simulink model "main_quad_rev5_31_315pm"  (R2023a)
settings: Solver=FixedStepAuto  StartTime=0.0  StopTime=inf  FixedStep=0.005  RelTol=1e-3
libraries: canmsglib x16, speedgoatlib_IO691 x12, slrealtimeutilitieslib x8
(part 1 of 2)
settings Model: SimulationMode=external  NumberOfSteps=2  ExtModeEnableFloating=off  Creator=celwe  LastModifiedBy=johna
settings SolverCC: ConcurrentTasks=on  PositivePriorityOrder=on
settings OptimizationCC: BlockReduction=off  OptimizeBlockIOStorage=off
settings DebuggingCC: TasksWithSamePriorityMsg=none  UnconnectedInputMsg=warning  UnconnectedOutputMsg=warning  UnconnectedLineMsg=warning
settings HardwareCC: ProdBitPerLong=64  ProdLongLongMode=on  ProdHWDeviceType=Intel->x86-64 (Linux 64)
settings ModelReferenceCC: EnableRefExpFcnMdlSchedulingChecks=on
settings RTWCC: Description=Simulink Real-Time  SystemTargetFile=slrealtime.tlc  TemplateMakefile=slrealtime_default_tmf  Toolchain=Simulink Real-Time Toolchain  BuildConfiguration=Faster Runs  CodeExecutionProfiling=on  TargetLang=C++  DLArmComputeVersion=19.05

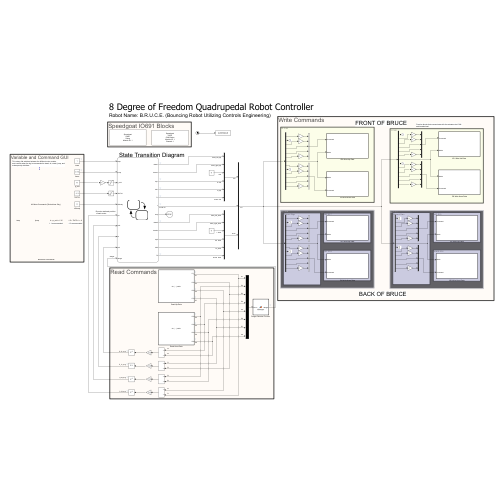
[thumbnail: Simulink's stored preview of the top-level diagram]
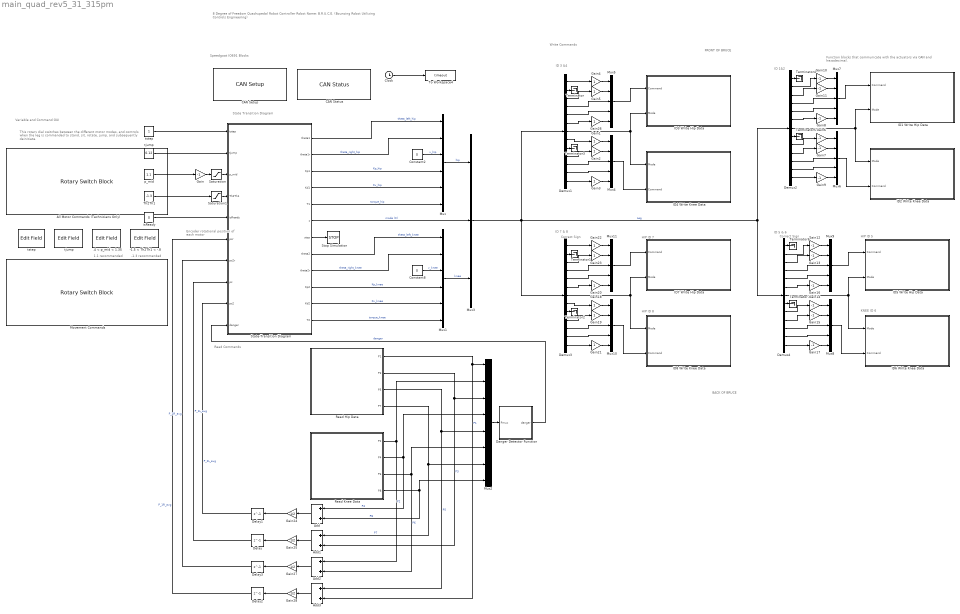
== system main_quad_rev5_31_315pm ==
  note: Variable and Command GUI
  note: 8 Degree of Freedom Quadrupedal Robot Controller
      | Robot Name: B.R.U.C.E. (Bouncing Robot Utilizing Controls Engineering)
  note: Encoder rotational position
      |  of each motor
  note: This rotary dial switches between the different motor modes,
      | and controls when the leg is commanded to stand, sit, rotate, jump, and
      | subsequently deinitiate.
  note: ID 1&2
  note: ID 3 &4
  note: BACK OF BRUCE
  note: HIP ID 5
  note: HIP ID 8
  note: KNEE ID 6
  note: ID 5 & 6
  note: FRONT OF BRUCE
  note: ID 7 & 8
  note: HIP ID 7
  note: Function blocks that communicate with the actuators via CAN
      | and hexadecimal.
  note: Correct Sign
  note: Correct Sign
  note: -1.3 recommended
  note: 1.1 recommended
  note: Speedgoat IO691 Blocks
  note: Read Commands
  note: Write Commands
  note: State Transition Diagram
  " tjump " : Constant  Value=0.12
  " tstep " : Constant
  -1.5 < Th2Th1 < -.8 : EditField  LabelPosition=Hide  ShowInitialText=on  Alignment=Center
  .4 < p_mid < 1.35 : EditField  LabelPosition=Hide  ShowInitialText=on  Alignment=Center
  Add{,1..3} (4 alike) : Sum
  "All Motor Commands (Technicians Only) " : RotarySwitchBlock
      settings: Values={{'Zeroing', 'Initiated', 'Stand', 'Sit', 'Right Up', 'Left Up', 'Jump', 'PrepJump', 'deinit'}, [0 1 2 3 5 6 7 8 4]}
  "CAN Setup " : speedgoatlib_IO691/Legacy/CAN Setup   moduletype=IO691  id=1  pciSlot=-1  chn1=CAN (HS)  chn2=CAN (HS)  chn3=Disabled  chn4=Disabled  initStruct=[]  termStruct=[]  ArbitrationbdrChn1=1.0 MBaud  ArbitrationManbdrChn1=[2,8,31,8]  FdbdrChn1=5.0 MBaud  FdManbdrChn1=[2,2,5,2]  ArbitrationbdrChn2=1.0 MBaud  ArbitrationManbdrChn2=[2,8,31,8]  FdbdrChn2=5.0 MBaud  FdManbdrChn2=[2,2,5,2]  ArbitrationbdrChn3=1.0 MBaud  ArbitrationManbdrChn3=[2,8,31,8]  FdbdrChn3=5.0 MBaud  FdManbdrChn3=[2,2,5,2]  ArbitrationbdrChn4=1.0 MBaud  ArbitrationManbdrChn4=[2,8,31,8]  FdbdrChn4=5.0 MBaud  FdManbdrChn4=[2,2,5,2]  moduleInitValues=[691 1 -1 -1]
      settings: SourceProductName=Simulink Real-Time: Speedgoat I/O Blockset
  CAN Status : speedgoatlib_IO691/Legacy/CAN Status  moduleId=1  sampleTime=-1  channel=1  busRecovery=Off  arrayOutput=off  controllerCpuLoad=off  controllerLiveCount=off  initModeAct=off  avgBusLoad=off  receiving=off  RxQueueEmpty=off  dataOverrunRcv=off  rxBufferLevel=off  txPending=off  dataOverrunTx=off  txBufferLevel=off  errWarnLimit=off  errPassLimit=off  errBusOff=off  busRecoveryCounter=off  busCouplingErr=off  transceiverErr=off  opMode=off  brp=off  timeSegment1=off  timeSegment2=off  synchronisationJumpWidth=off  dataTSEG1=off  dataTSEG2=off  dataSJW=off  moduleType=691  qtyStatBlk=1  ptIdx=0  isFDMod=0
      settings: SourceProductName=Simulink Real-Time: Speedgoat I/O Blockset
  Clock : Clock
  Constant2 : Constant  Value=0
  Constant8 : Constant  Value=0
  Danger Detector Function : MATLAB Function  TreatAsAtomicUnit=on
  Delay{,1..3} (4 alike) : Delay  DelayLength=1
  Demux{1..4} (4 alike) : Demux  Outputs=13
  Gain{,6..17} (13 alike) : Gain  Gain=-1
  Gain{1..5,18..23,26} (12 alike) : Gain
  Gain{24..25,27..28} (4 alike) : Gain  Gain=1/2
  ID1 Write Hip Data : Subsystem  TreatAsAtomicUnit=on
  ID2 Write Knee Data : Subsystem  TreatAsAtomicUnit=on
  ID3 Write Hip Data : Subsystem  TreatAsAtomicUnit=on
  ID4 Write Knee Data : Subsystem  TreatAsAtomicUnit=on
  ID5 Write Hip Data : Subsystem  TreatAsAtomicUnit=on
  ID6 Write Knee Data : Subsystem  TreatAsAtomicUnit=on
  ID7 Write Hip Data : Subsystem  TreatAsAtomicUnit=on
  ID8 Write Knee Data : Subsystem  TreatAsAtomicUnit=on
  Movement Commands : RotarySwitchBlock
      settings: Values={{'Stand', 'Sit', 'Right Up', 'Left Up', 'Jump', 'Prep Jump'}, [2 3 5 6 7 8]}
  Mux : Mux  Inputs=6
  Mux1 : Mux  Inputs=6
  Mux{4..11} (8 alike) : Mux  Inputs=5
  Mux2 : Mux  Inputs=8
  Mux3 : Mux  Inputs=3
  Read Hip Data : Subsystem  TreatAsAtomicUnit=on
  Read Knee Data : Subsystem  TreatAsAtomicUnit=on
  Saturation : Saturate  UpperLimit=-.4  LowerLimit=-1.35
  Saturation1 : Saturate  UpperLimit=-.8  LowerLimit=-1.5
  State-Transition Diagram : Stateflow chart  TreatAsAtomicUnit=on
      settings: PortSchema="{\"entries\":[{\"content\":{\"sides\":[{\"content\":{\"connectorIds\":[\"In7\",\"In8\",\"In9\",\"In10\",\"In4\",\"In5\",\"In6\",\"In1\",\"In2\",\"In3\"]},\"type\":\"ConnectorPlacement.EquallySpacedRectSide\",\"uuid\":\"09499f21-f50c-4ce4-914e-8b9942bcc246\"},{\"content\":{\"connectorIds\":[\"Out2\",\"Out11\",\"Out7\",\"Out9\",\"Out5\",\"Out4\",\"Out1\",\"Out3\",\"Out12\",\"Out8\",\"Out10\",\"Out6\"],\"side\":\"RIGHT\"},\"type\":\"ConnectorPlacement.EquallySpacedRectSide\",\"uuid\":\"b935e908-ace3-4dfb-ad6d-08dfed6ffdb3\"},{\"content\":{\"connectorIds\":[],\"side\":\"TOP\"},\"type\":\"ConnectorPlacement.EquallySpacedRectSide\",\"uuid\":\"4cd7c5d6-1f1f-4a1f-84b4-9b198395645e\"}]},\"type\":\"ConnectorPlacement.EquallySpacedConnector\",\"uuid\":\"2dc6a8af-05a8-4f21-87ab-6863f156f450\"}],\"packageUris\":[\"http://schema.mathworks.com/mf0/Connector/R2020b\"],\"version\":\"1.0\"}"
  Stop Simulation : Stop
  Terminator{,1..7} (8 alike) : Terminator
  Th2Th1 : Constant  Value=-1.3
  To Workspace4 : ToWorkspace  VariableName=timeout  SampleTime=-1
  isReady : Constant  Value=0
  p_mid : Constant  Value=1.1
  tjump : EditField  LabelPosition=Hide  ShowInitialText=on  Alignment=Center
  tstep : EditField  LabelPosition=Hide  ShowInitialText=on  Alignment=Center
  wires:
  Mux/1 -> Mux3/1  "hip"
  State-Transition Diagram/7(Kp1) -> Mux/4  "Kp_hip"
  State-Transition Diagram/5(T1) -> Mux/6  "torque_hip"
  Constant8/1 -> Mux1/3  "v_knee"
  Mux1/1 -> Mux3/3  "knee"
  State-Transition Diagram/4(c) -> Mux3/2  "mode (C)"
  Mux2/1 -> Danger Detector Function/1(Pmux)
  Danger Detector Function/1(danger) -> State-Transition Diagram/3(danger)  "danger"
  Delay/1 -> State-Transition Diagram/1(pc)  "P_1L_avg"
  State-Transition Diagram/1(stop) -> Stop Simulation/1
  Delay1/1 -> State-Transition Diagram/2(pc2)  "P_2L_avg"
  isReady/1 -> State-Transition Diagram/4(isReady)
  Clock/1 -> To Workspace4/1
  State-Transition Diagram/9(Kd1) -> Mux/5  "Kv_hip"
  Constant2/1 -> Mux/3  "v_hip"
  State-Transition Diagram/2(theta1) -> Mux/1  "theta_left_hip"
  Mux11/1 -> ID7 Write Hip Data/1(Command)
  Mux10/1 -> ID8 Write Knee Data/2(Command)
  Mux3/1 -> Demux3/1, Demux4/1, Demux2/1, Demux1/1  "Leg"
  Gain24/1 -> Delay1/1
  Gain25/1 -> Delay/1
  Add/1 -> Gain24/1
  Add1/1 -> Gain25/1
  Mux9/1 -> ID5 Write Hip Data/1(Command)
  Mux8/1 -> ID6 Write Knee Data/2(Command)
  Mux7/1 -> ID1 Write Hip Data/1(Command)
  Mux6/1 -> ID2 Write Knee Data/2(Command)
  Demux1/8 -> Gain1/1
  Demux1/5 -> Mux5/4
  Demux1/7 -> ID4 Write Knee Data/1(Mode), ID3 Write Hip Data/2(Mode)
  Demux1/12 -> Mux4/4
  Gain3/1 -> Mux4/5
  Gain1/1 -> Mux4/1
  Gain2/1 -> Mux4/2
  Mux5/1 -> ID3 Write Hip Data/1(Command)
  Gain4/1 -> Mux5/1
  Gain5/1 -> Mux5/2
  Mux4/1 -> ID4 Write Knee Data/2(Command)
  Demux1/6 -> Gain26/1
  Demux1/11 -> Mux4/3
  Gain26/1 -> Mux5/5
  Demux1/3 -> Gain5/1
  Demux1/10 -> Gain2/1
  Demux1/1 -> Gain4/1
  Demux1/4 -> Mux5/3
  Read Knee Data/1(P2) -> Add2/1, Mux2/2  "P2"
  Read Knee Data/2(P4) -> Add/1, Mux2/4  "P4"
  Read Knee Data/3(P6) -> Add2/2, Mux2/6  "P6"
  Read Knee Data/4(P8) -> Add/2, Mux2/8  "P8"
  Read Hip Data/4(P7) -> Add1/1, Mux2/7  "P7"
  Read Hip Data/3(P5) -> Add3/1, Mux2/5  "P5"
  Read Hip Data/2(P3) -> Add1/2, Mux2/3  "P3"
  Read Hip Data/1(P1) -> Add3/2, Mux2/1  "P1"
  Gain28/1 -> Delay2/1
  Gain27/1 -> Delay3/1
  Add2/1 -> Gain27/1
  Add3/1 -> Gain28/1
  Delay3/1 -> State-Transition Diagram/6(pc2r)  "P_2R_avg"
  Delay2/1 -> State-Transition Diagram/5(pcr)  "P_1R_avg"
  State-Transition Diagram/11(theta1r) -> Mux/2  "theta_right_hip"
  Demux1/13 -> Gain3/1
  Demux2/7 -> ID1 Write Hip Data/2(Mode), ID2 Write Knee Data/1(Mode)
  Demux2/4 -> Mux7/3
  Demux2/10 -> Gain7/1
  Demux2/6 -> Gain8/1
  Demux2/5 -> Mux7/4
  Demux2/11 -> Mux6/3
  Demux2/3 -> Gain11/1
  Demux2/12 -> Mux6/4
  Gain11/1 -> Mux7/2
  Gain10/1 -> Mux7/1
  Gain7/1 -> Mux6/2
  Demux2/13 -> Gain9/1
  Gain9/1 -> Mux6/5
  Gain8/1 -> Mux7/5
  Gain6/1 -> Mux6/1
  Demux2/2 -> Gain10/1
  Demux2/9 -> Gain6/1
  Demux3/7 -> ID7 Write Hip Data/2(Mode), ID8 Write Knee Data/1(Mode)
  Demux3/4 -> Mux11/3
  Demux3/10 -> Gain19/1
  Demux3/6 -> Gain20/1
  Demux3/5 -> Mux11/4
  Demux3/11 -> Mux10/3
  Demux3/3 -> Gain23/1
  Demux3/12 -> Mux10/4
  Gain23/1 -> Mux11/2
  Demux3/1 -> Gain22/1
  Gain22/1 -> Mux11/1
  Gain19/1 -> Mux10/2
  Demux3/13 -> Gain21/1
  Gain21/1 -> Mux10/5
  Demux3/8 -> Gain18/1
  Gain20/1 -> Mux11/5
  Gain18/1 -> Mux10/1
  Demux4/5 -> Mux9/4
  Demux4/6 -> Gain16/1
  Demux4/10 -> Gain15/1
  Demux4/7 -> ID6 Write Knee Data/1(Mode), ID5 Write Hip Data/2(Mode)
  Demux4/2 -> Gain12/1
  Demux4/3 -> Gain13/1
  Demux4/9 -> Gain14/1
  Demux4/11 -> Mux8/3
  Gain12/1 -> Mux9/1
  Gain13/1 -> Mux9/2
  Gain17/1 -> Mux8/5
  Demux4/13 -> Gain17/1
  Gain14/1 -> Mux8/1
  Gain15/1 -> Mux8/2
  Demux4/12 -> Mux8/4
  Gain16/1 -> Mux9/5
  Demux4/4 -> Mux9/3
  Demux1/2 -> Terminator/1
  Demux3/2 -> Terminator1/1
  Demux3/9 -> Terminator2/1
  Demux1/9 -> Terminator3/1
  Demux2/1 -> Terminator4/1
  Demux2/8 -> Terminator5/1
  Demux4/1 -> Terminator6/1
  Demux4/8 -> Terminator7/1
  State-Transition Diagram/12(theta2r) -> Mux1/2  "theta_right_knee"
  State-Transition Diagram/3(theta2) -> Mux1/1  "theta_left_knee"
  State-Transition Diagram/10(Kd2) -> Mux1/5  "Kv_knee"
  State-Transition Diagram/6(T2) -> Mux1/6  "torque_knee"
  State-Transition Diagram/8(Kp2) -> Mux1/4  "Kp_knee"
  " tjump "/1 -> State-Transition Diagram/8(tjump)
  " tstep "/1 -> State-Transition Diagram/7(tstep)
  p_mid/1 -> Gain/1
  Saturation/1 -> State-Transition Diagram/9(p_mid)
  Gain/1 -> Saturation/1
  Th2Th1/1 -> Saturation1/1
  Saturation1/1 -> State-Transition Diagram/10(Th2Th1)

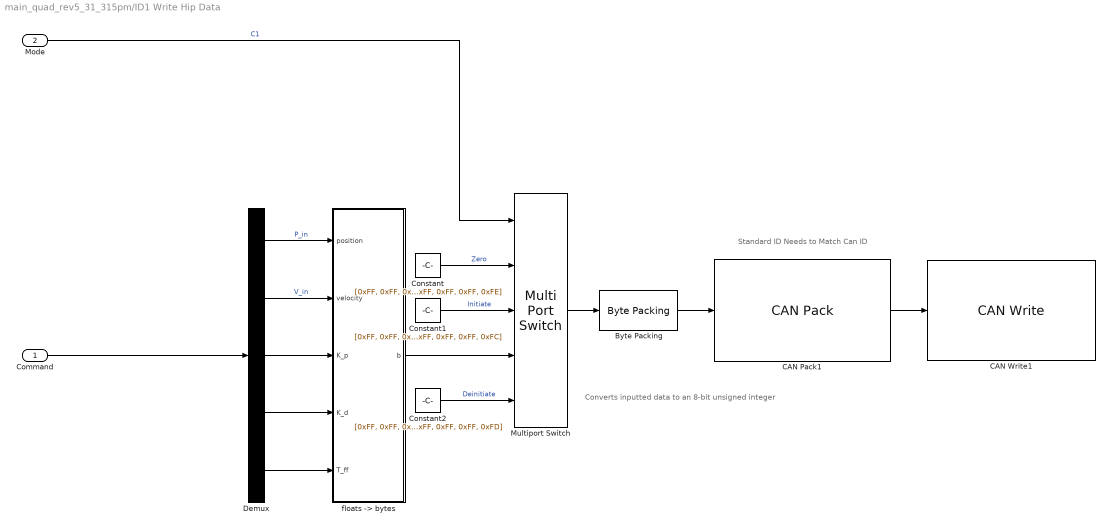
== system main_quad_rev5_31_315pm/ID1 Write Hip Data ==
  note: Standard ID Needs to Match Can ID
  note: Converts inputted data to an 8-bit unsigned integer
  Command : Inport
  Mode : Inport  Port=2
  Byte Packing : slrealtimeutilitieslib/Byte Packing  MaskPackedDataType=uint8  MaskUnpackedDataTypes={['uint8']}  MaskAlignment=1
  CAN Pack1 : canmsglib/CAN Pack  MsgList=(none)  MsgName=CAN Msg  MsgIDType=Standard (11-bit identifier)  MsgIdentifier=1  MsgLength=8  Remote=off  ApplyMinMax=off  BusOutput=off  SignalInfo={ 'b1', '0', '8', 'LE', 'unsigned', 'Standard', '0', '1', '0', '-Inf', 'Inf'; 'b2', '8', '8', 'LE', 'unsigned', 'Standard', '0', '1', '0', '-Inf', 'Inf'; 'b3', '16', '8', 'LE', 'unsigned', 'Standard', '0', '1', '0', '-Inf', 'Inf'; 'b4', '24', '8', 'LE', 'unsigned', 'Standard', '0', '1', '0', '-Inf', 'Inf'; 'b5', '32', '8', 'LE', 'unsigned', 'Standard', '0', '1', '0', '-Inf', 'Inf'; 'b6', '40', '8', 'LE', 'unsigned', 'Standard', '0', '1', '0', '-Inf', 'Inf'; 'b7', '48', '8', 'LE', 'unsigned', 'Standard', '0', '1', '0', '-Inf', 'Inf'; 'b8', '56', '8', 'LE', 'unsigned', 'Standard', '0', '1', '0', '-Inf', 'Inf' }
      settings: DataFormat=raw data
  CAN Write1 : speedgoatlib_IO691/Legacy/CAN Write  id=1  ts=-1  channel=1  messageType=CAN  BusInput=off  enableStatusPort=off  canType=CAN (HS)  initValues=[691 1 -1 0 1 1 0 0]
      settings: SourceProductName=Simulink Real-Time: Speedgoat I/O Blockset
  Constant : Constant  Value=[0xFF, 0xFF, 0xFF, 0xFF, 0xFF, 0xFF, 0xFF, 0xFE]
  Constant1 : Constant  Value=[0xFF, 0xFF, 0xFF, 0xFF, 0xFF, 0xFF, 0xFF, 0xFC]
  Constant2 : Constant  Value=[0xFF, 0xFF, 0xFF, 0xFF, 0xFF, 0xFF, 0xFF, 0xFD]
  Demux : Demux  Outputs=5
  Multiport Switch : MultiPortSwitch  Inputs=4  DiagnosticForDefault=None  SaturateOnIntegerOverflow=off  InputSameDT=off
  "floats -> bytes" : MATLAB Function  TreatAsAtomicUnit=on
  wires:
  Demux/5 -> "floats -> bytes"/5(T_ff)
  Multiport Switch/1 -> Byte Packing/1
  Demux/4 -> "floats -> bytes"/4(K_d)
  Demux/1 -> "floats -> bytes"/1(position)  "P_in"
  Constant/1 -> Multiport Switch/2  "Zero"
  Demux/2 -> "floats -> bytes"/2(velocity)  "V_in"
  Constant2/1 -> Multiport Switch/5  "Deinitiate"
  CAN Pack1/1 -> CAN Write1/1
  Byte Packing/1 -> CAN Pack1/1
  Constant1/1 -> Multiport Switch/3  "Initiate"
  "floats -> bytes"/1(b) -> Multiport Switch/4
  Demux/3 -> "floats -> bytes"/3(K_p)
  Mode/1 -> Multiport Switch/1  "C1"
  Command/1 -> Demux/1

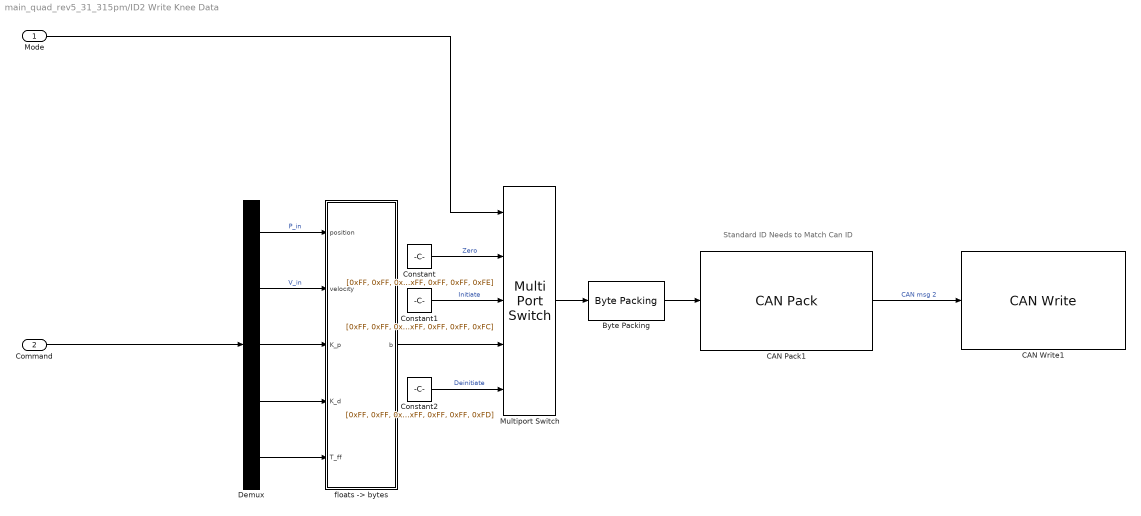
== system main_quad_rev5_31_315pm/ID2 Write Knee Data ==
  note: Standard ID Needs to Match Can ID
  Mode : Inport
  Command : Inport  Port=2
  Byte Packing : slrealtimeutilitieslib/Byte Packing  MaskPackedDataType=uint8  MaskUnpackedDataTypes={['uint8']}  MaskAlignment=1
  CAN Pack1 : canmsglib/CAN Pack  MsgList=(none)  MsgName=CAN Msg  MsgIDType=Standard (11-bit identifier)  MsgIdentifier=2  MsgLength=8  Remote=off  ApplyMinMax=off  BusOutput=off  SignalInfo={ 'b1', '0', '8', 'LE', 'unsigned', 'Standard', '0', '1', '0', '-Inf', 'Inf'; 'b2', '8', '8', 'LE', 'unsigned', 'Standard', '0', '1', '0', '-Inf', 'Inf'; 'b3', '16', '8', 'LE', 'unsigned', 'Standard', '0', '1', '0', '-Inf', 'Inf'; 'b4', '24', '8', 'LE', 'unsigned', 'Standard', '0', '1', '0', '-Inf', 'Inf'; 'b5', '32', '8', 'LE', 'unsigned', 'Standard', '0', '1', '0', '-Inf', 'Inf'; 'b6', '40', '8', 'LE', 'unsigned', 'Standard', '0', '1', '0', '-Inf', 'Inf'; 'b7', '48', '8', 'LE', 'unsigned', 'Standard', '0', '1', '0', '-Inf', 'Inf'; 'b8', '56', '8', 'LE', 'unsigned', 'Standard', '0', '1', '0', '-Inf', 'Inf' }
      settings: DataFormat=raw data
  CAN Write1 : speedgoatlib_IO691/Legacy/CAN Write  id=1  ts=-1  channel=2  messageType=CAN  BusInput=off  enableStatusPort=off  canType=CAN (HS)  initValues=[691 1 -1 1 1 1 0 0]
      settings: SourceProductName=Simulink Real-Time: Speedgoat I/O Blockset
  Constant : Constant  Value=[0xFF, 0xFF, 0xFF, 0xFF, 0xFF, 0xFF, 0xFF, 0xFE]
  Constant1 : Constant  Value=[0xFF, 0xFF, 0xFF, 0xFF, 0xFF, 0xFF, 0xFF, 0xFC]
  Constant2 : Constant  Value=[0xFF, 0xFF, 0xFF, 0xFF, 0xFF, 0xFF, 0xFF, 0xFD]
  Demux : Demux  Outputs=5
  Multiport Switch : MultiPortSwitch  Inputs=4  DiagnosticForDefault=None  SaturateOnIntegerOverflow=off  InputSameDT=off
  "floats -> bytes" : MATLAB Function  TreatAsAtomicUnit=on
  wires:
  Demux/5 -> "floats -> bytes"/5(T_ff)
  Multiport Switch/1 -> Byte Packing/1
  Demux/4 -> "floats -> bytes"/4(K_d)
  Demux/1 -> "floats -> bytes"/1(position)  "P_in"
  Constant/1 -> Multiport Switch/2  "Zero"
  Demux/2 -> "floats -> bytes"/2(velocity)  "V_in"
  Constant2/1 -> Multiport Switch/5  "Deinitiate"
  CAN Pack1/1 -> CAN Write1/1  "CAN msg 2"
  Byte Packing/1 -> CAN Pack1/1
  Constant1/1 -> Multiport Switch/3  "Initiate"
  "floats -> bytes"/1(b) -> Multiport Switch/4
  Demux/3 -> "floats -> bytes"/3(K_p)
  Mode/1 -> Multiport Switch/1
  Command/1 -> Demux/1

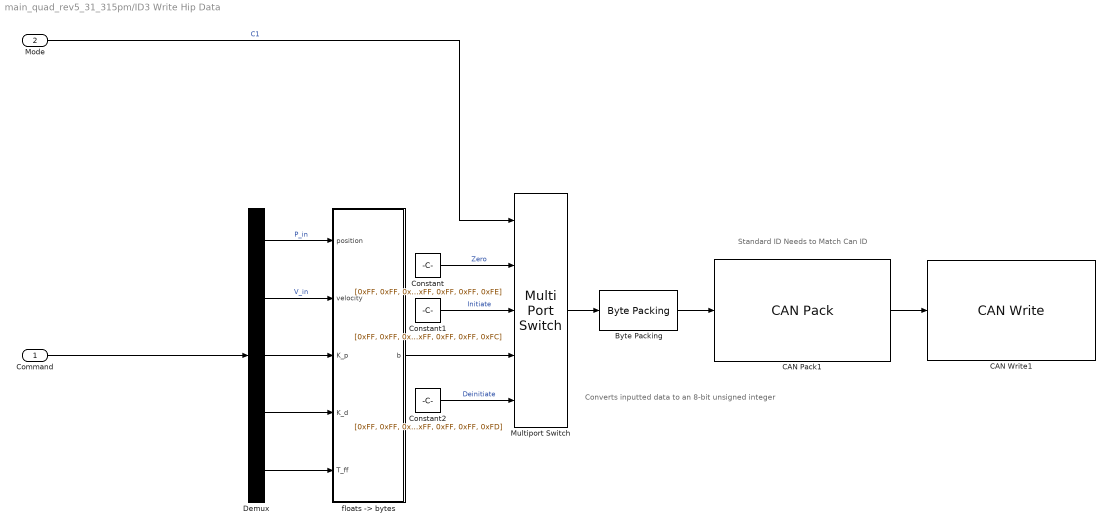
== system main_quad_rev5_31_315pm/ID3 Write Hip Data ==
  note: Standard ID Needs to Match Can ID
  note: Converts inputted data to an 8-bit unsigned integer
  Command : Inport
  Mode : Inport  Port=2
  Byte Packing : slrealtimeutilitieslib/Byte Packing  MaskPackedDataType=uint8  MaskUnpackedDataTypes={['uint8']}  MaskAlignment=1
  CAN Pack1 : canmsglib/CAN Pack  MsgList=(none)  MsgName=CAN Msg  MsgIDType=Standard (11-bit identifier)  MsgIdentifier=3  MsgLength=8  Remote=off  ApplyMinMax=off  BusOutput=off  SignalInfo={ 'b1', '0', '8', 'LE', 'unsigned', 'Standard', '0', '1', '0', '-Inf', 'Inf'; 'b2', '8', '8', 'LE', 'unsigned', 'Standard', '0', '1', '0', '-Inf', 'Inf'; 'b3', '16', '8', 'LE', 'unsigned', 'Standard', '0', '1', '0', '-Inf', 'Inf'; 'b4', '24', '8', 'LE', 'unsigned', 'Standard', '0', '1', '0', '-Inf', 'Inf'; 'b5', '32', '8', 'LE', 'unsigned', 'Standard', '0', '1', '0', '-Inf', 'Inf'; 'b6', '40', '8', 'LE', 'unsigned', 'Standard', '0', '1', '0', '-Inf', 'Inf'; 'b7', '48', '8', 'LE', 'unsigned', 'Standard', '0', '1', '0', '-Inf', 'Inf'; 'b8', '56', '8', 'LE', 'unsigned', 'Standard', '0', '1', '0', '-Inf', 'Inf' }
      settings: DataFormat=raw data
  CAN Write1 : speedgoatlib_IO691/Legacy/CAN Write  id=1  ts=-1  channel=1  messageType=CAN  BusInput=off  enableStatusPort=off  canType=CAN (HS)  initValues=[691 1 -1 0 1 1 0 0]
      settings: SourceProductName=Simulink Real-Time: Speedgoat I/O Blockset
  Constant : Constant  Value=[0xFF, 0xFF, 0xFF, 0xFF, 0xFF, 0xFF, 0xFF, 0xFE]
  Constant1 : Constant  Value=[0xFF, 0xFF, 0xFF, 0xFF, 0xFF, 0xFF, 0xFF, 0xFC]
  Constant2 : Constant  Value=[0xFF, 0xFF, 0xFF, 0xFF, 0xFF, 0xFF, 0xFF, 0xFD]
  Demux : Demux  Outputs=5
  Multiport Switch : MultiPortSwitch  Inputs=4  DiagnosticForDefault=None  SaturateOnIntegerOverflow=off  InputSameDT=off
  "floats -> bytes" : MATLAB Function  TreatAsAtomicUnit=on
  wires:
  Demux/5 -> "floats -> bytes"/5(T_ff)
  Multiport Switch/1 -> Byte Packing/1
  Demux/4 -> "floats -> bytes"/4(K_d)
  Demux/1 -> "floats -> bytes"/1(position)  "P_in"
  Constant/1 -> Multiport Switch/2  "Zero"
  Demux/2 -> "floats -> bytes"/2(velocity)  "V_in"
  Constant2/1 -> Multiport Switch/5  "Deinitiate"
  CAN Pack1/1 -> CAN Write1/1
  Byte Packing/1 -> CAN Pack1/1
  Constant1/1 -> Multiport Switch/3  "Initiate"
  "floats -> bytes"/1(b) -> Multiport Switch/4
  Demux/3 -> "floats -> bytes"/3(K_p)
  Mode/1 -> Multiport Switch/1  "C1"
  Command/1 -> Demux/1

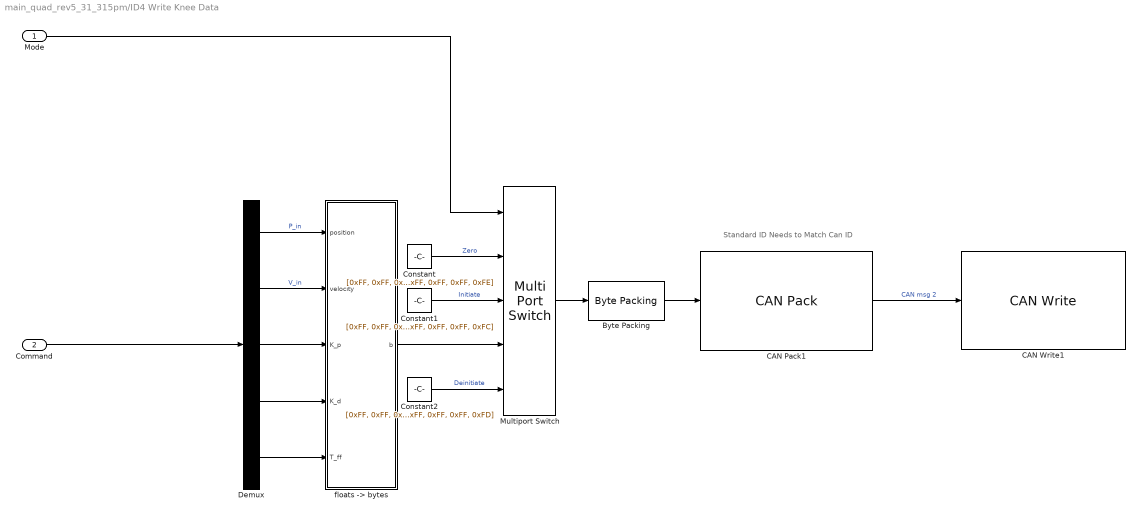
== system main_quad_rev5_31_315pm/ID4 Write Knee Data ==
  note: Standard ID Needs to Match Can ID
  Mode : Inport
  Command : Inport  Port=2
  Byte Packing : slrealtimeutilitieslib/Byte Packing  MaskPackedDataType=uint8  MaskUnpackedDataTypes={['uint8']}  MaskAlignment=1
  CAN Pack1 : canmsglib/CAN Pack  MsgList=(none)  MsgName=CAN Msg  MsgIDType=Standard (11-bit identifier)  MsgIdentifier=4  MsgLength=8  Remote=off  ApplyMinMax=off  BusOutput=off  SignalInfo={ 'b1', '0', '8', 'LE', 'unsigned', 'Standard', '0', '1', '0', '-Inf', 'Inf'; 'b2', '8', '8', 'LE', 'unsigned', 'Standard', '0', '1', '0', '-Inf', 'Inf'; 'b3', '16', '8', 'LE', 'unsigned', 'Standard', '0', '1', '0', '-Inf', 'Inf'; 'b4', '24', '8', 'LE', 'unsigned', 'Standard', '0', '1', '0', '-Inf', 'Inf'; 'b5', '32', '8', 'LE', 'unsigned', 'Standard', '0', '1', '0', '-Inf', 'Inf'; 'b6', '40', '8', 'LE', 'unsigned', 'Standard', '0', '1', '0', '-Inf', 'Inf'; 'b7', '48', '8', 'LE', 'unsigned', 'Standard', '0', '1', '0', '-Inf', 'Inf'; 'b8', '56', '8', 'LE', 'unsigned', 'Standard', '0', '1', '0', '-Inf', 'Inf' }
      settings: DataFormat=raw data
  CAN Write1 : speedgoatlib_IO691/Legacy/CAN Write  id=1  ts=-1  channel=2  messageType=CAN  BusInput=off  enableStatusPort=off  canType=CAN (HS)  initValues=[691 1 -1 1 1 1 0 0]
      settings: SourceProductName=Simulink Real-Time: Speedgoat I/O Blockset
  Constant : Constant  Value=[0xFF, 0xFF, 0xFF, 0xFF, 0xFF, 0xFF, 0xFF, 0xFE]
  Constant1 : Constant  Value=[0xFF, 0xFF, 0xFF, 0xFF, 0xFF, 0xFF, 0xFF, 0xFC]
  Constant2 : Constant  Value=[0xFF, 0xFF, 0xFF, 0xFF, 0xFF, 0xFF, 0xFF, 0xFD]
  Demux : Demux  Outputs=5
  Multiport Switch : MultiPortSwitch  Inputs=4  DiagnosticForDefault=None  SaturateOnIntegerOverflow=off  InputSameDT=off
  "floats -> bytes" : MATLAB Function  TreatAsAtomicUnit=on
  wires:
  Demux/5 -> "floats -> bytes"/5(T_ff)
  Multiport Switch/1 -> Byte Packing/1
  Demux/4 -> "floats -> bytes"/4(K_d)
  Demux/1 -> "floats -> bytes"/1(position)  "P_in"
  Constant/1 -> Multiport Switch/2  "Zero"
  Demux/2 -> "floats -> bytes"/2(velocity)  "V_in"
  Constant2/1 -> Multiport Switch/5  "Deinitiate"
  CAN Pack1/1 -> CAN Write1/1  "CAN msg 2"
  Byte Packing/1 -> CAN Pack1/1
  Constant1/1 -> Multiport Switch/3  "Initiate"
  "floats -> bytes"/1(b) -> Multiport Switch/4
  Demux/3 -> "floats -> bytes"/3(K_p)
  Mode/1 -> Multiport Switch/1
  Command/1 -> Demux/1

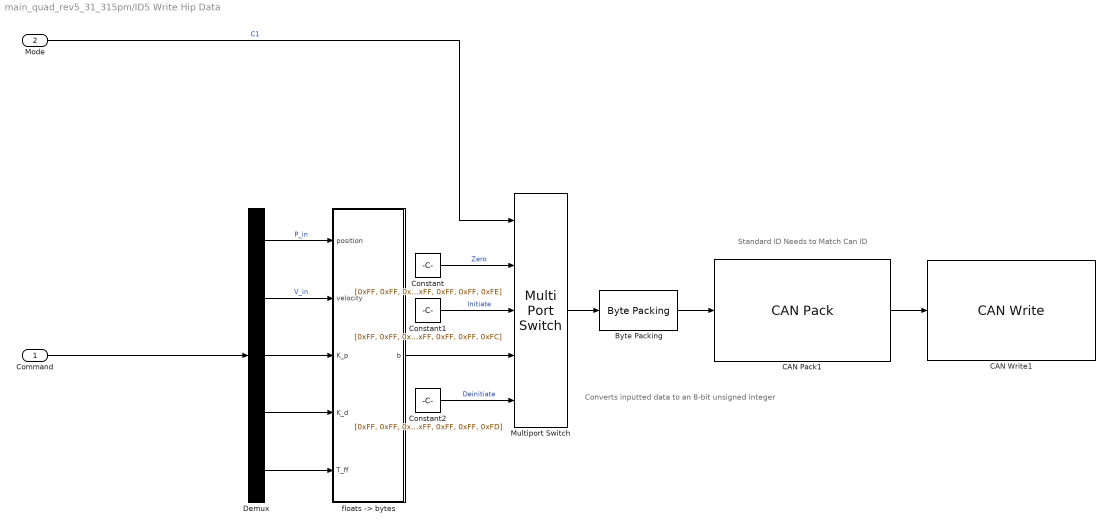
== system main_quad_rev5_31_315pm/ID5 Write Hip Data ==
  note: Standard ID Needs to Match Can ID
  note: Converts inputted data to an 8-bit unsigned integer
  Command : Inport
  Mode : Inport  Port=2
  Byte Packing : slrealtimeutilitieslib/Byte Packing  MaskPackedDataType=uint8  MaskUnpackedDataTypes={['uint8']}  MaskAlignment=1
  CAN Pack1 : canmsglib/CAN Pack  MsgList=(none)  MsgName=CAN Msg  MsgIDType=Standard (11-bit identifier)  MsgIdentifier=5  MsgLength=8  Remote=off  ApplyMinMax=off  BusOutput=off  SignalInfo={ 'b1', '0', '8', 'LE', 'unsigned', 'Standard', '0', '1', '0', '-Inf', 'Inf'; 'b2', '8', '8', 'LE', 'unsigned', 'Standard', '0', '1', '0', '-Inf', 'Inf'; 'b3', '16', '8', 'LE', 'unsigned', 'Standard', '0', '1', '0', '-Inf', 'Inf'; 'b4', '24', '8', 'LE', 'unsigned', 'Standard', '0', '1', '0', '-Inf', 'Inf'; 'b5', '32', '8', 'LE', 'unsigned', 'Standard', '0', '1', '0', '-Inf', 'Inf'; 'b6', '40', '8', 'LE', 'unsigned', 'Standard', '0', '1', '0', '-Inf', 'Inf'; 'b7', '48', '8', 'LE', 'unsigned', 'Standard', '0', '1', '0', '-Inf', 'Inf'; 'b8', '56', '8', 'LE', 'unsigned', 'Standard', '0', '1', '0', '-Inf', 'Inf' }
      settings: DataFormat=raw data
  CAN Write1 : speedgoatlib_IO691/Legacy/CAN Write  id=1  ts=-1  channel=1  messageType=CAN  BusInput=off  enableStatusPort=off  canType=CAN (HS)  initValues=[691 1 -1 0 1 1 0 0]
      settings: SourceProductName=Simulink Real-Time: Speedgoat I/O Blockset
  Constant : Constant  Value=[0xFF, 0xFF, 0xFF, 0xFF, 0xFF, 0xFF, 0xFF, 0xFE]
  Constant1 : Constant  Value=[0xFF, 0xFF, 0xFF, 0xFF, 0xFF, 0xFF, 0xFF, 0xFC]
  Constant2 : Constant  Value=[0xFF, 0xFF, 0xFF, 0xFF, 0xFF, 0xFF, 0xFF, 0xFD]
  Demux : Demux  Outputs=5
  Multiport Switch : MultiPortSwitch  Inputs=4  DiagnosticForDefault=None  SaturateOnIntegerOverflow=off  InputSameDT=off
  "floats -> bytes" : MATLAB Function  TreatAsAtomicUnit=on
  wires:
  Demux/5 -> "floats -> bytes"/5(T_ff)
  Multiport Switch/1 -> Byte Packing/1
  Demux/4 -> "floats -> bytes"/4(K_d)
  Demux/1 -> "floats -> bytes"/1(position)  "P_in"
  Constant/1 -> Multiport Switch/2  "Zero"
  Demux/2 -> "floats -> bytes"/2(velocity)  "V_in"
  Constant2/1 -> Multiport Switch/5  "Deinitiate"
  CAN Pack1/1 -> CAN Write1/1
  Byte Packing/1 -> CAN Pack1/1
  Constant1/1 -> Multiport Switch/3  "Initiate"
  "floats -> bytes"/1(b) -> Multiport Switch/4
  Demux/3 -> "floats -> bytes"/3(K_p)
  Mode/1 -> Multiport Switch/1  "C1"
  Command/1 -> Demux/1

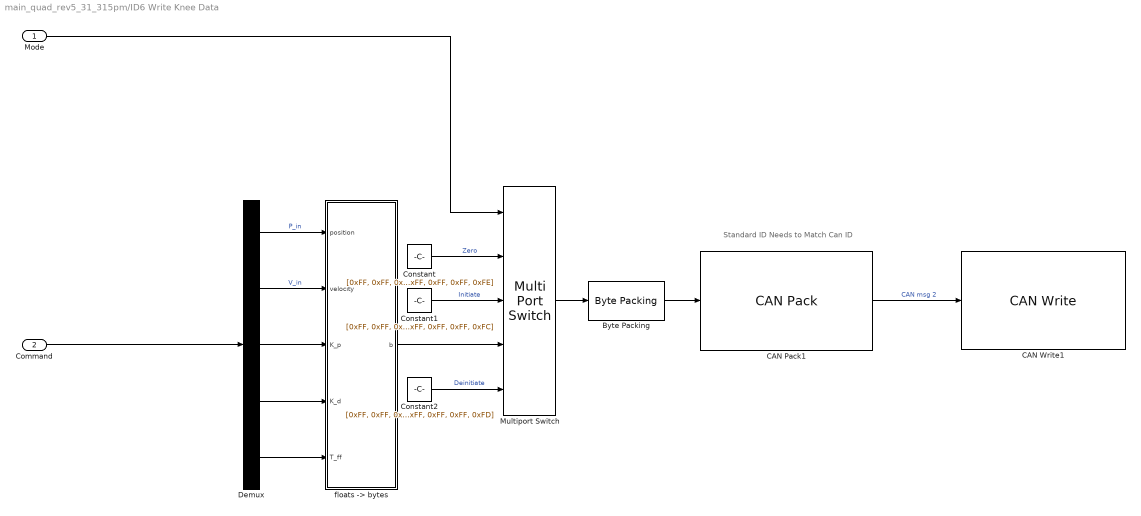
== system main_quad_rev5_31_315pm/ID6 Write Knee Data ==
  note: Standard ID Needs to Match Can ID
  Mode : Inport
  Command : Inport  Port=2
  Byte Packing : slrealtimeutilitieslib/Byte Packing  MaskPackedDataType=uint8  MaskUnpackedDataTypes={['uint8']}  MaskAlignment=1
  CAN Pack1 : canmsglib/CAN Pack  MsgList=(none)  MsgName=CAN Msg  MsgIDType=Standard (11-bit identifier)  MsgIdentifier=6  MsgLength=8  Remote=off  ApplyMinMax=off  BusOutput=off  SignalInfo={ 'b1', '0', '8', 'LE', 'unsigned', 'Standard', '0', '1', '0', '-Inf', 'Inf'; 'b2', '8', '8', 'LE', 'unsigned', 'Standard', '0', '1', '0', '-Inf', 'Inf'; 'b3', '16', '8', 'LE', 'unsigned', 'Standard', '0', '1', '0', '-Inf', 'Inf'; 'b4', '24', '8', 'LE', 'unsigned', 'Standard', '0', '1', '0', '-Inf', 'Inf'; 'b5', '32', '8', 'LE', 'unsigned', 'Standard', '0', '1', '0', '-Inf', 'Inf'; 'b6', '40', '8', 'LE', 'unsigned', 'Standard', '0', '1', '0', '-Inf', 'Inf'; 'b7', '48', '8', 'LE', 'unsigned', 'Standard', '0', '1', '0', '-Inf', 'Inf'; 'b8', '56', '8', 'LE', 'unsigned', 'Standard', '0', '1', '0', '-Inf', 'Inf' }
      settings: DataFormat=raw data
  CAN Write1 : speedgoatlib_IO691/Legacy/CAN Write  id=1  ts=-1  channel=2  messageType=CAN  BusInput=off  enableStatusPort=off  canType=CAN (HS)  initValues=[691 1 -1 1 1 1 0 0]
      settings: SourceProductName=Simulink Real-Time: Speedgoat I/O Blockset
  Constant : Constant  Value=[0xFF, 0xFF, 0xFF, 0xFF, 0xFF, 0xFF, 0xFF, 0xFE]
  Constant1 : Constant  Value=[0xFF, 0xFF, 0xFF, 0xFF, 0xFF, 0xFF, 0xFF, 0xFC]
  Constant2 : Constant  Value=[0xFF, 0xFF, 0xFF, 0xFF, 0xFF, 0xFF, 0xFF, 0xFD]
  Demux : Demux  Outputs=5
  Multiport Switch : MultiPortSwitch  Inputs=4  DiagnosticForDefault=None  SaturateOnIntegerOverflow=off  InputSameDT=off
  "floats -> bytes" : MATLAB Function  TreatAsAtomicUnit=on
  wires:
  Demux/5 -> "floats -> bytes"/5(T_ff)
  Multiport Switch/1 -> Byte Packing/1
  Demux/4 -> "floats -> bytes"/4(K_d)
  Demux/1 -> "floats -> bytes"/1(position)  "P_in"
  Constant/1 -> Multiport Switch/2  "Zero"
  Demux/2 -> "floats -> bytes"/2(velocity)  "V_in"
  Constant2/1 -> Multiport Switch/5  "Deinitiate"
  CAN Pack1/1 -> CAN Write1/1  "CAN msg 2"
  Byte Packing/1 -> CAN Pack1/1
  Constant1/1 -> Multiport Switch/3  "Initiate"
  "floats -> bytes"/1(b) -> Multiport Switch/4
  Demux/3 -> "floats -> bytes"/3(K_p)
  Mode/1 -> Multiport Switch/1
  Command/1 -> Demux/1

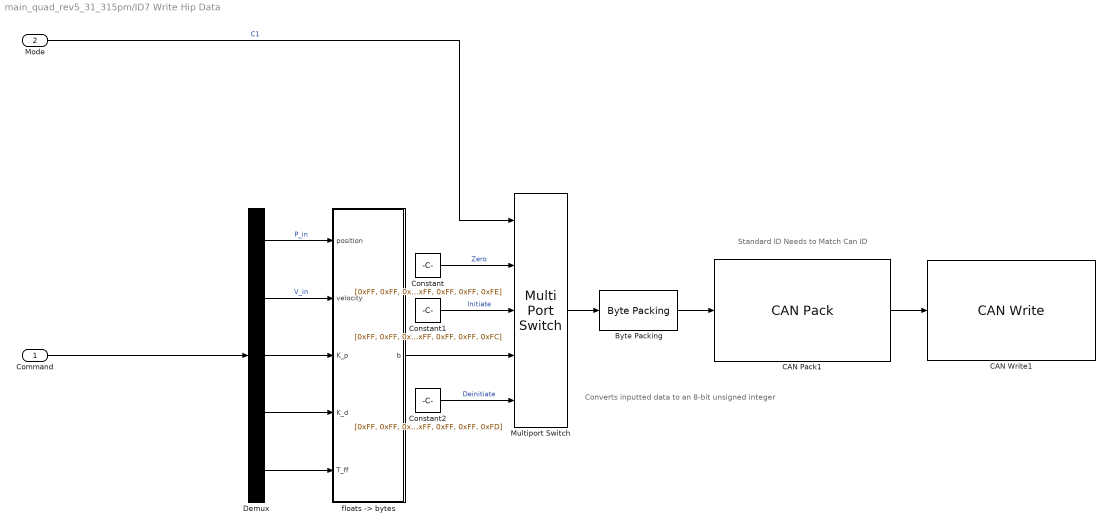
== system main_quad_rev5_31_315pm/ID7 Write Hip Data ==
  note: Standard ID Needs to Match Can ID
  note: Converts inputted data to an 8-bit unsigned integer
  Command : Inport
  Mode : Inport  Port=2
  Byte Packing : slrealtimeutilitieslib/Byte Packing  MaskPackedDataType=uint8  MaskUnpackedDataTypes={['uint8']}  MaskAlignment=1
  CAN Pack1 : canmsglib/CAN Pack  MsgList=(none)  MsgName=CAN Msg  MsgIDType=Standard (11-bit identifier)  MsgIdentifier=7  MsgLength=8  Remote=off  ApplyMinMax=off  BusOutput=off  SignalInfo={ 'b1', '0', '8', 'LE', 'unsigned', 'Standard', '0', '1', '0', '-Inf', 'Inf'; 'b2', '8', '8', 'LE', 'unsigned', 'Standard', '0', '1', '0', '-Inf', 'Inf'; 'b3', '16', '8', 'LE', 'unsigned', 'Standard', '0', '1', '0', '-Inf', 'Inf'; 'b4', '24', '8', 'LE', 'unsigned', 'Standard', '0', '1', '0', '-Inf', 'Inf'; 'b5', '32', '8', 'LE', 'unsigned', 'Standard', '0', '1', '0', '-Inf', 'Inf'; 'b6', '40', '8', 'LE', 'unsigned', 'Standard', '0', '1', '0', '-Inf', 'Inf'; 'b7', '48', '8', 'LE', 'unsigned', 'Standard', '0', '1', '0', '-Inf', 'Inf'; 'b8', '56', '8', 'LE', 'unsigned', 'Standard', '0', '1', '0', '-Inf', 'Inf' }
      settings: DataFormat=raw data
  CAN Write1 : speedgoatlib_IO691/Legacy/CAN Write  id=1  ts=-1  channel=1  messageType=CAN  BusInput=off  enableStatusPort=off  canType=CAN (HS)  initValues=[691 1 -1 0 1 1 0 0]
      settings: SourceProductName=Simulink Real-Time: Speedgoat I/O Blockset
  Constant : Constant  Value=[0xFF, 0xFF, 0xFF, 0xFF, 0xFF, 0xFF, 0xFF, 0xFE]
  Constant1 : Constant  Value=[0xFF, 0xFF, 0xFF, 0xFF, 0xFF, 0xFF, 0xFF, 0xFC]
  Constant2 : Constant  Value=[0xFF, 0xFF, 0xFF, 0xFF, 0xFF, 0xFF, 0xFF, 0xFD]
  Demux : Demux  Outputs=5
  Multiport Switch : MultiPortSwitch  Inputs=4  DiagnosticForDefault=None  SaturateOnIntegerOverflow=off  InputSameDT=off
  "floats -> bytes" : MATLAB Function  TreatAsAtomicUnit=on
  wires:
  Demux/5 -> "floats -> bytes"/5(T_ff)
  Multiport Switch/1 -> Byte Packing/1
  Demux/4 -> "floats -> bytes"/4(K_d)
  Demux/1 -> "floats -> bytes"/1(position)  "P_in"
  Constant/1 -> Multiport Switch/2  "Zero"
  Demux/2 -> "floats -> bytes"/2(velocity)  "V_in"
  Constant2/1 -> Multiport Switch/5  "Deinitiate"
  CAN Pack1/1 -> CAN Write1/1
  Byte Packing/1 -> CAN Pack1/1
  Constant1/1 -> Multiport Switch/3  "Initiate"
  "floats -> bytes"/1(b) -> Multiport Switch/4
  Demux/3 -> "floats -> bytes"/3(K_p)
  Mode/1 -> Multiport Switch/1  "C1"
  Command/1 -> Demux/1

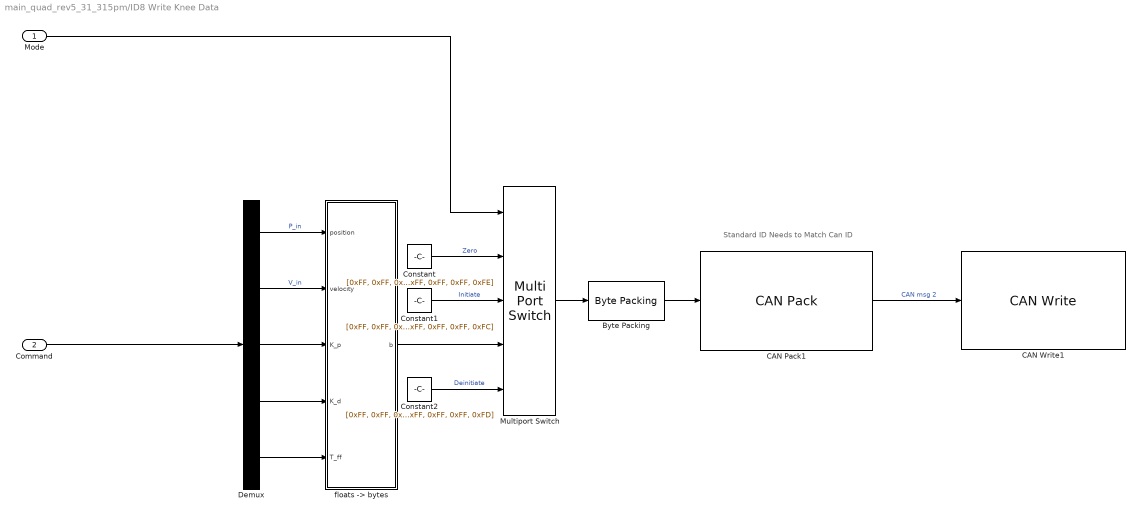
== system main_quad_rev5_31_315pm/ID8 Write Knee Data ==
  note: Standard ID Needs to Match Can ID
  Mode : Inport
  Command : Inport  Port=2
  Byte Packing : slrealtimeutilitieslib/Byte Packing  MaskPackedDataType=uint8  MaskUnpackedDataTypes={['uint8']}  MaskAlignment=1
  CAN Pack1 : canmsglib/CAN Pack  MsgList=(none)  MsgName=CAN Msg  MsgIDType=Standard (11-bit identifier)  MsgIdentifier=8  MsgLength=8  Remote=off  ApplyMinMax=off  BusOutput=off  SignalInfo={ 'b1', '0', '8', 'LE', 'unsigned', 'Standard', '0', '1', '0', '-Inf', 'Inf'; 'b2', '8', '8', 'LE', 'unsigned', 'Standard', '0', '1', '0', '-Inf', 'Inf'; 'b3', '16', '8', 'LE', 'unsigned', 'Standard', '0', '1', '0', '-Inf', 'Inf'; 'b4', '24', '8', 'LE', 'unsigned', 'Standard', '0', '1', '0', '-Inf', 'Inf'; 'b5', '32', '8', 'LE', 'unsigned', 'Standard', '0', '1', '0', '-Inf', 'Inf'; 'b6', '40', '8', 'LE', 'unsigned', 'Standard', '0', '1', '0', '-Inf', 'Inf'; 'b7', '48', '8', 'LE', 'unsigned', 'Standard', '0', '1', '0', '-Inf', 'Inf'; 'b8', '56', '8', 'LE', 'unsigned', 'Standard', '0', '1', '0', '-Inf', 'Inf' }
      settings: DataFormat=raw data
  CAN Write1 : speedgoatlib_IO691/Legacy/CAN Write  id=1  ts=-1  channel=2  messageType=CAN  BusInput=off  enableStatusPort=off  canType=CAN (HS)  initValues=[691 1 -1 1 1 1 0 0]
      settings: SourceProductName=Simulink Real-Time: Speedgoat I/O Blockset
  Constant : Constant  Value=[0xFF, 0xFF, 0xFF, 0xFF, 0xFF, 0xFF, 0xFF, 0xFE]
  Constant1 : Constant  Value=[0xFF, 0xFF, 0xFF, 0xFF, 0xFF, 0xFF, 0xFF, 0xFC]
  Constant2 : Constant  Value=[0xFF, 0xFF, 0xFF, 0xFF, 0xFF, 0xFF, 0xFF, 0xFD]
  Demux : Demux  Outputs=5
  Multiport Switch : MultiPortSwitch  Inputs=4  DiagnosticForDefault=None  SaturateOnIntegerOverflow=off  InputSameDT=off
  "floats -> bytes" : MATLAB Function  TreatAsAtomicUnit=on
  wires:
  Demux/5 -> "floats -> bytes"/5(T_ff)
  Multiport Switch/1 -> Byte Packing/1
  Demux/4 -> "floats -> bytes"/4(K_d)
  Demux/1 -> "floats -> bytes"/1(position)  "P_in"
  Constant/1 -> Multiport Switch/2  "Zero"
  Demux/2 -> "floats -> bytes"/2(velocity)  "V_in"
  Constant2/1 -> Multiport Switch/5  "Deinitiate"
  CAN Pack1/1 -> CAN Write1/1  "CAN msg 2"
  Byte Packing/1 -> CAN Pack1/1
  Constant1/1 -> Multiport Switch/3  "Initiate"
  "floats -> bytes"/1(b) -> Multiport Switch/4
  Demux/3 -> "floats -> bytes"/3(K_p)
  Mode/1 -> Multiport Switch/1
  Command/1 -> Demux/1

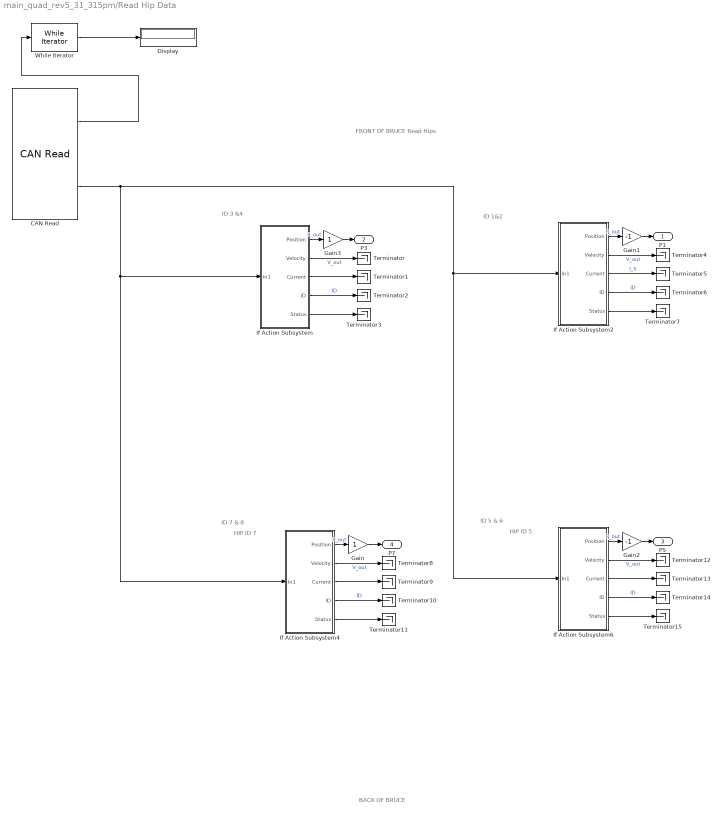
== system main_quad_rev5_31_315pm/Read Hip Data ==
  note: HIP ID 5
  note: FRONT OF BRUCE
      | Read Hips
  note: ID 7 & 8
  note: ID 5 & 6
  note: ID 1&2
  note: ID 3 &4
  note: HIP ID 7
  note: BACK OF BRUCE
  CAN Read : speedgoatlib_IO691/Legacy/CAN Read  id=1  ts=-1  channel=1  messageType=CAN  canType=CAN (HS)  BusOutput=off  initValues=[691 1 -1 0 1 1 0]
      settings: SourceProductName=Simulink Real-Time: Speedgoat I/O Blockset
  Display : Display
  Gain : Gain
  Gain1 : Gain  Gain=-1
  Gain2 : Gain  Gain=-1
  Gain3 : Gain
  If Action Subsystem : Subsystem  TreatAsAtomicUnit=on
  If Action Subsystem2 : Subsystem  TreatAsAtomicUnit=on
  If Action Subsystem4 : Subsystem  TreatAsAtomicUnit=on
  If Action Subsystem6 : Subsystem  TreatAsAtomicUnit=on
  Terminator{,1..15} (16 alike) : Terminator
  While Iterator : WhileIterator  MaxIters=-1  WhileBlockType=do-while  ResetStates=reset  ShowIterationPort=on
  P1 : Outport
  P3 : Outport  Port=2
  P5 : Outport  Port=3
  P7 : Outport  Port=4
  wires:
  CAN Read/1 -> While Iterator/1
  If Action Subsystem/1(Position) -> Gain3/1  "P_out"
  While Iterator/1 -> Display/1
  If Action Subsystem2/1(Position) -> Gain1/1  "P_out"
  If Action Subsystem4/1(Position) -> Gain/1  "P_out"
  If Action Subsystem6/1(Position) -> Gain2/1  "P_out"
  CAN Read/2 -> If Action Subsystem2/1(In1), If Action Subsystem6/1(In1), If Action Subsystem4/1(In1), If Action Subsystem/1(In1)
  Gain2/1 -> P5/1
  Gain1/1 -> P1/1
  Gain/1 -> P7/1
  Gain3/1 -> P3/1
  If Action Subsystem/2(Velocity) -> Terminator/1  "V_out"
  If Action Subsystem/3(Current) -> Terminator1/1
  If Action Subsystem/4(ID) -> Terminator2/1  "ID"
  If Action Subsystem/5(Status) -> Terminator3/1
  If Action Subsystem2/5(Status) -> Terminator7/1
  If Action Subsystem2/4(ID) -> Terminator6/1  "ID"
  If Action Subsystem2/2(Velocity) -> Terminator4/1  "V_out"
  If Action Subsystem2/3(Current) -> Terminator5/1  "I_5"
  If Action Subsystem4/5(Status) -> Terminator11/1
  If Action Subsystem4/4(ID) -> Terminator10/1  "ID"
  If Action Subsystem4/2(Velocity) -> Terminator8/1  "V_out"
  If Action Subsystem4/3(Current) -> Terminator9/1
  If Action Subsystem6/5(Status) -> Terminator15/1
  If Action Subsystem6/4(ID) -> Terminator14/1  "ID"
  If Action Subsystem6/2(Velocity) -> Terminator12/1  "V_out"
  If Action Subsystem6/3(Current) -> Terminator13/1

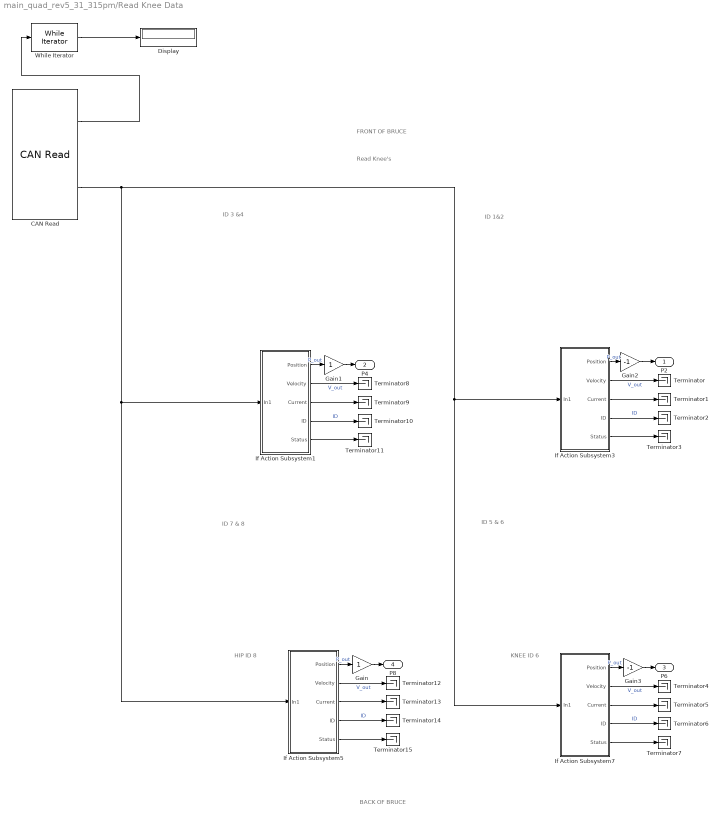
== system main_quad_rev5_31_315pm/Read Knee Data ==
  note: FRONT OF BRUCE
  note: ID 7 & 8
  note: ID 5 & 6
  note: ID 1&2
  note: ID 3 &4
  note: KNEE ID 6
  note: HIP ID 8
  note: BACK OF BRUCE
  note: Read Knee's
  CAN Read : speedgoatlib_IO691/Legacy/CAN Read  id=1  ts=-1  channel=2  messageType=CAN  canType=CAN (HS)  BusOutput=off  initValues=[691 1 -1 1 1 1 0]
      settings: SourceProductName=Simulink Real-Time: Speedgoat I/O Blockset
  Display : Display
  Gain : Gain
  Gain1 : Gain
  Gain2 : Gain  Gain=-1
  Gain3 : Gain  Gain=-1
  If Action Subsystem1 : Subsystem  TreatAsAtomicUnit=on
  If Action Subsystem3 : Subsystem  TreatAsAtomicUnit=on
  If Action Subsystem5 : Subsystem  TreatAsAtomicUnit=on
  If Action Subsystem7 : Subsystem  TreatAsAtomicUnit=on
  Terminator{,1..15} (16 alike) : Terminator
  While Iterator : WhileIterator  MaxIters=-1  WhileBlockType=do-while  ResetStates=reset  ShowIterationPort=on
  P2 : Outport
  P4 : Outport  Port=2
  P6 : Outport  Port=3
  P8 : Outport  Port=4
  wires:
  CAN Read/1 -> While Iterator/1
  While Iterator/1 -> Display/1
  If Action Subsystem1/1(Position) -> Gain1/1  "P_out"
  If Action Subsystem3/1(Position) -> Gain2/1  "P_out"
  If Action Subsystem5/1(Position) -> Gain/1  "P_out"
  If Action Subsystem7/1(Position) -> Gain3/1  "P_out"
  CAN Read/2 -> If Action Subsystem7/1(In1), If Action Subsystem3/1(In1), If Action Subsystem5/1(In1), If Action Subsystem1/1(In1)
  Gain/1 -> P8/1
  Gain1/1 -> P4/1
  Gain2/1 -> P2/1
  Gain3/1 -> P6/1
  If Action Subsystem3/5(Status) -> Terminator3/1
  If Action Subsystem3/4(ID) -> Terminator2/1  "ID"
  If Action Subsystem3/2(Velocity) -> Terminator/1  "V_out"
  If Action Subsystem3/3(Current) -> Terminator1/1
  If Action Subsystem7/5(Status) -> Terminator7/1
  If Action Subsystem7/4(ID) -> Terminator6/1  "ID"
  If Action Subsystem7/2(Velocity) -> Terminator4/1  "V_out"
  If Action Subsystem7/3(Current) -> Terminator5/1
  If Action Subsystem1/5(Status) -> Terminator11/1
  If Action Subsystem1/4(ID) -> Terminator10/1  "ID"
  If Action Subsystem1/2(Velocity) -> Terminator8/1  "V_out"
  If Action Subsystem1/3(Current) -> Terminator9/1
  If Action Subsystem5/5(Status) -> Terminator15/1
  If Action Subsystem5/4(ID) -> Terminator14/1  "ID"
  If Action Subsystem5/2(Velocity) -> Terminator12/1  "V_out"
  If Action Subsystem5/3(Current) -> Terminator13/1

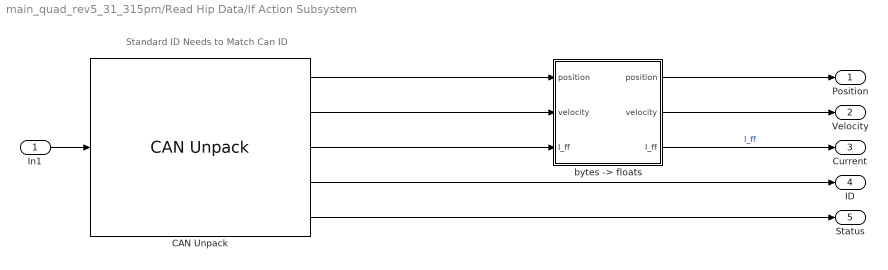
== system main_quad_rev5_31_315pm/Read Hip Data/If Action Subsystem ==
  note: Standard ID Needs to Match Can ID
  In1 : Inport
  CAN Unpack : canmsglib/CAN Unpack  MsgList=(none)  MsgName=CAN Msg  MsgIDType=Standard (11-bit identifier)  MsgIdentifier=3  MsgLength=6  SignalInfo={ 'position', '16', '16', 'BE', 'unsigned', 'Standard', '0', '1', '0', '0', '65535'; 'velocity', '36', '12', 'BE', 'unsigned', 'Standard', '0', '1', '0', '0', '4095'; 'current', '40', '12', 'BE', 'unsigned', 'Standard', '0', '1', '0', '0', '4095'; 'id', '0', '8', 'BE', 'unsigned', 'Standard', '0', '1', '0', '0', '255' }  IDPort=off  TimestampPort=off  ErrorPort=off  RemotePort=off  LengthPort=off  StatusPort=on  ApplyMinMax=off
  "bytes -> floats" : MATLAB Function  TreatAsAtomicUnit=on
  Position : Outport
  Velocity : Outport  Port=2
  Current : Outport  Port=3
  ID : Outport  Port=4
  Status : Outport  Port=5
  wires:
  CAN Unpack/5 -> Status/1
  CAN Unpack/3 -> "bytes -> floats"/3("I_ff ")
  CAN Unpack/4 -> ID/1
  "bytes -> floats"/2(velocity) -> Velocity/1
  "bytes -> floats"/3(I_ff) -> Current/1  "I_ff"
  CAN Unpack/2 -> "bytes -> floats"/2("velocity ")
  In1/1 -> CAN Unpack/1
  CAN Unpack/1 -> "bytes -> floats"/1("position ")
  "bytes -> floats"/1(position) -> Position/1

== system main_quad_rev5_31_315pm/Read Hip Data/If Action Subsystem2 ==
  note: Standard ID Needs to Match Can ID
  In1 : Inport
  CAN Unpack : canmsglib/CAN Unpack  MsgList=(none)  MsgName=CAN Msg  MsgIDType=Standard (11-bit identifier)  MsgIdentifier=1  MsgLength=6  SignalInfo={ 'position', '16', '16', 'BE', 'unsigned', 'Standard', '0', '1', '0', '0', '65535'; 'velocity', '36', '12', 'BE', 'unsigned', 'Standard', '0', '1', '0', '0', '4095'; 'current', '40', '12', 'BE', 'unsigned', 'Standard', '0', '1', '0', '0', '4095'; 'id', '0', '8', 'BE', 'unsigned', 'Standard', '0', '1', '0', '0', '255' }  IDPort=off  TimestampPort=off  ErrorPort=off  RemotePort=off  LengthPort=off  StatusPort=on  ApplyMinMax=off
  "bytes -> floats" : MATLAB Function  TreatAsAtomicUnit=on
  Position : Outport
  Velocity : Outport  Port=2
  Current : Outport  Port=3
  ID : Outport  Port=4
  Status : Outport  Port=5
  wires:
  CAN Unpack/5 -> Status/1
  CAN Unpack/3 -> "bytes -> floats"/3("I_ff ")
  CAN Unpack/4 -> ID/1
  "bytes -> floats"/2(velocity) -> Velocity/1
  "bytes -> floats"/3(I_ff) -> Current/1
  CAN Unpack/2 -> "bytes -> floats"/2("velocity ")
  In1/1 -> CAN Unpack/1
  CAN Unpack/1 -> "bytes -> floats"/1("position ")
  "bytes -> floats"/1(position) -> Position/1

== system main_quad_rev5_31_315pm/Read Hip Data/If Action Subsystem4 ==
  note: Standard ID Needs to Match Can ID
  In1 : Inport
  CAN Unpack : canmsglib/CAN Unpack  MsgList=(none)  MsgName=CAN Msg  MsgIDType=Standard (11-bit identifier)  MsgIdentifier=7  MsgLength=6  SignalInfo={ 'position', '16', '16', 'BE', 'unsigned', 'Standard', '0', '1', '0', '0', '65535'; 'velocity', '36', '12', 'BE', 'unsigned', 'Standard', '0', '1', '0', '0', '4095'; 'current', '40', '12', 'BE', 'unsigned', 'Standard', '0', '1', '0', '0', '4095'; 'id', '0', '8', 'BE', 'unsigned', 'Standard', '0', '1', '0', '0', '255' }  IDPort=off  TimestampPort=off  ErrorPort=off  RemotePort=off  LengthPort=off  StatusPort=on  ApplyMinMax=off
  "bytes -> floats" : MATLAB Function  TreatAsAtomicUnit=on
  Position : Outport
  Velocity : Outport  Port=2
  Current : Outport  Port=3
  ID : Outport  Port=4
  Status : Outport  Port=5
  wires:
  CAN Unpack/5 -> Status/1
  CAN Unpack/3 -> "bytes -> floats"/3("I_ff ")
  CAN Unpack/4 -> ID/1
  "bytes -> floats"/2(velocity) -> Velocity/1
  "bytes -> floats"/3(I_ff) -> Current/1  "I_ff"
  CAN Unpack/2 -> "bytes -> floats"/2("velocity ")
  In1/1 -> CAN Unpack/1
  CAN Unpack/1 -> "bytes -> floats"/1("position ")
  "bytes -> floats"/1(position) -> Position/1

== system main_quad_rev5_31_315pm/Read Hip Data/If Action Subsystem6 ==
  note: Standard ID Needs to Match Can ID
  In1 : Inport
  CAN Unpack : canmsglib/CAN Unpack  MsgList=(none)  MsgName=CAN Msg  MsgIDType=Standard (11-bit identifier)  MsgIdentifier=5  MsgLength=6  SignalInfo={ 'position', '16', '16', 'BE', 'unsigned', 'Standard', '0', '1', '0', '0', '65535'; 'velocity', '36', '12', 'BE', 'unsigned', 'Standard', '0', '1', '0', '0', '4095'; 'current', '40', '12', 'BE', 'unsigned', 'Standard', '0', '1', '0', '0', '4095'; 'id', '0', '8', 'BE', 'unsigned', 'Standard', '0', '1', '0', '0', '255' }  IDPort=off  TimestampPort=off  ErrorPort=off  RemotePort=off  LengthPort=off  StatusPort=on  ApplyMinMax=off
  "bytes -> floats" : MATLAB Function  TreatAsAtomicUnit=on
  Position : Outport
  Velocity : Outport  Port=2
  Current : Outport  Port=3
  ID : Outport  Port=4
  Status : Outport  Port=5
  wires:
  CAN Unpack/5 -> Status/1
  CAN Unpack/3 -> "bytes -> floats"/3("I_ff ")
  CAN Unpack/4 -> ID/1
  "bytes -> floats"/2(velocity) -> Velocity/1
  "bytes -> floats"/3(I_ff) -> Current/1  "I_ff"
  CAN Unpack/2 -> "bytes -> floats"/2("velocity ")
  In1/1 -> CAN Unpack/1
  CAN Unpack/1 -> "bytes -> floats"/1("position ")
  "bytes -> floats"/1(position) -> Position/1

== system main_quad_rev5_31_315pm/Read Knee Data/If Action Subsystem1 ==
  note: Standard ID Needs to Match Can ID
  In1 : Inport
  CAN Unpack : canmsglib/CAN Unpack  MsgList=(none)  MsgName=CAN Msg  MsgIDType=Standard (11-bit identifier)  MsgIdentifier=4  MsgLength=6  SignalInfo={ 'position', '16', '16', 'BE', 'unsigned', 'Standard', '0', '1', '0', '0', '65535'; 'velocity', '36', '12', 'BE', 'unsigned', 'Standard', '0', '1', '0', '0', '4095'; 'current', '40', '12', 'BE', 'unsigned', 'Standard', '0', '1', '0', '0', '4095'; 'id', '0', '8', 'BE', 'unsigned', 'Standard', '0', '1', '0', '0', '255' }  IDPort=off  TimestampPort=off  ErrorPort=off  RemotePort=off  LengthPort=off  StatusPort=on  ApplyMinMax=off
  "bytes -> floats" : MATLAB Function  TreatAsAtomicUnit=on
  Position : Outport
  Velocity : Outport  Port=2
  Current : Outport  Port=3
  ID : Outport  Port=4
  Status : Outport  Port=5
  wires:
  CAN Unpack/5 -> Status/1
  CAN Unpack/1 -> "bytes -> floats"/1("position ")
  CAN Unpack/3 -> "bytes -> floats"/3("I_ff ")
  "bytes -> floats"/1(position) -> Position/1
  CAN Unpack/4 -> ID/1
  "bytes -> floats"/2(velocity) -> Velocity/1
  "bytes -> floats"/3(I_ff) -> Current/1  "I_ff"
  CAN Unpack/2 -> "bytes -> floats"/2("velocity ")
  In1/1 -> CAN Unpack/1

== system main_quad_rev5_31_315pm/Read Knee Data/If Action Subsystem3 ==
  note: Standard ID Needs to Match Can ID
  In1 : Inport
  CAN Unpack : canmsglib/CAN Unpack  MsgList=(none)  MsgName=CAN Msg  MsgIDType=Standard (11-bit identifier)  MsgIdentifier=2  MsgLength=6  SignalInfo={ 'position', '16', '16', 'BE', 'unsigned', 'Standard', '0', '1', '0', '0', '65535'; 'velocity', '36', '12', 'BE', 'unsigned', 'Standard', '0', '1', '0', '0', '4095'; 'current', '40', '12', 'BE', 'unsigned', 'Standard', '0', '1', '0', '0', '4095'; 'id', '0', '8', 'BE', 'unsigned', 'Standard', '0', '1', '0', '0', '255' }  IDPort=off  TimestampPort=off  ErrorPort=off  RemotePort=off  LengthPort=off  StatusPort=on  ApplyMinMax=off
  "bytes -> floats" : MATLAB Function  TreatAsAtomicUnit=on
  Position : Outport
  Velocity : Outport  Port=2
  Current : Outport  Port=3
  ID : Outport  Port=4
  Status : Outport  Port=5
  wires:
  CAN Unpack/5 -> Status/1
  CAN Unpack/1 -> "bytes -> floats"/1("position ")
  CAN Unpack/3 -> "bytes -> floats"/3("I_ff ")
  "bytes -> floats"/1(position) -> Position/1
  CAN Unpack/4 -> ID/1
  "bytes -> floats"/2(velocity) -> Velocity/1
  "bytes -> floats"/3(I_ff) -> Current/1  "I_ff"
  CAN Unpack/2 -> "bytes -> floats"/2("velocity ")
  In1/1 -> CAN Unpack/1

== system main_quad_rev5_31_315pm/Read Knee Data/If Action Subsystem5 ==
  note: Standard ID Needs to Match Can ID
  In1 : Inport
  CAN Unpack : canmsglib/CAN Unpack  MsgList=(none)  MsgName=CAN Msg  MsgIDType=Standard (11-bit identifier)  MsgIdentifier=8  MsgLength=6  SignalInfo={ 'position', '16', '16', 'BE', 'unsigned', 'Standard', '0', '1', '0', '0', '65535'; 'velocity', '36', '12', 'BE', 'unsigned', 'Standard', '0', '1', '0', '0', '4095'; 'current', '40', '12', 'BE', 'unsigned', 'Standard', '0', '1', '0', '0', '4095'; 'id', '0', '8', 'BE', 'unsigned', 'Standard', '0', '1', '0', '0', '255' }  IDPort=off  TimestampPort=off  ErrorPort=off  RemotePort=off  LengthPort=off  StatusPort=on  ApplyMinMax=off
  "bytes -> floats" : MATLAB Function  TreatAsAtomicUnit=on
  Position : Outport
  Velocity : Outport  Port=2
  Current : Outport  Port=3
  ID : Outport  Port=4
  Status : Outport  Port=5
  wires:
  CAN Unpack/5 -> Status/1
  CAN Unpack/1 -> "bytes -> floats"/1("position ")
  CAN Unpack/3 -> "bytes -> floats"/3("I_ff ")
  "bytes -> floats"/1(position) -> Position/1
  CAN Unpack/4 -> ID/1
  "bytes -> floats"/2(velocity) -> Velocity/1
  "bytes -> floats"/3(I_ff) -> Current/1  "I_ff"
  CAN Unpack/2 -> "bytes -> floats"/2("velocity ")
  In1/1 -> CAN Unpack/1

== system main_quad_rev5_31_315pm/Read Knee Data/If Action Subsystem7 ==
  note: Standard ID Needs to Match Can ID
  In1 : Inport
  CAN Unpack : canmsglib/CAN Unpack  MsgList=(none)  MsgName=CAN Msg  MsgIDType=Standard (11-bit identifier)  MsgIdentifier=6  MsgLength=6  SignalInfo={ 'position', '16', '16', 'BE', 'unsigned', 'Standard', '0', '1', '0', '0', '65535'; 'velocity', '36', '12', 'BE', 'unsigned', 'Standard', '0', '1', '0', '0', '4095'; 'current', '40', '12', 'BE', 'unsigned', 'Standard', '0', '1', '0', '0', '4095'; 'id', '0', '8', 'BE', 'unsigned', 'Standard', '0', '1', '0', '0', '255' }  IDPort=off  TimestampPort=off  ErrorPort=off  RemotePort=off  LengthPort=off  StatusPort=on  ApplyMinMax=off
  "bytes -> floats" : MATLAB Function  TreatAsAtomicUnit=on
  Position : Outport
  Velocity : Outport  Port=2
  Current : Outport  Port=3
  ID : Outport  Port=4
  Status : Outport  Port=5
  wires:
  CAN Unpack/5 -> Status/1
  CAN Unpack/1 -> "bytes -> floats"/1("position ")
  CAN Unpack/3 -> "bytes -> floats"/3("I_ff ")
  "bytes -> floats"/1(position) -> Position/1
  CAN Unpack/4 -> ID/1
  "bytes -> floats"/2(velocity) -> Velocity/1
  "bytes -> floats"/3(I_ff) -> Current/1  "I_ff"
  CAN Unpack/2 -> "bytes -> floats"/2("velocity ")
  In1/1 -> CAN Unpack/1

== matlab function main_quad_rev5_31_315pm/ID4 Write Knee Data/floats -> bytes ==
  data: position input; b output uint8 size=8; velocity input; K_p input; K_d input; T_ff input
function b = fcn(position, velocity, K_p, K_d, T_ff)

P_MIN  =-95.5;  % [rad]
P_MAX  = 95.5;  % [rad]
V_MIN  =-45;    % [rad/s] 30 to 45
V_MAX  = 45;    % [rad/s]
KP_MIN = 0;     % [Nm/rad]
KP_MAX = 500;   % [Nm/rad]
KD_MIN = 0;     % [Nm*s/rad
KD_MAX = 5;     % [Nm*s/rad
T_MIN  =-18;    % [Nm]
T_MAX  = 18;    % [Nm]

position = floor((max(min(position,P_MAX) ,P_MIN)  - P_MIN )*65535/(P_MAX  - P_MIN));
velocity = floor((max(min(velocity,V_MAX) ,V_MIN)  - V_MIN )*4095 /(V_MAX  - V_MIN));
K_p      = floor((max(min(K_p     ,KP_MAX),KP_MIN) - KP_MIN)*4095 /(KP_MAX - KP_MIN));
K_d      = floor((max(min(K_d     ,V_MAX) ,V_MIN)  - KD_MIN)*4095 /(KD_MAX - KD_MIN));
T_ff     = floor((max(min(T_ff    ,V_MAX) ,V_MIN)  - T_MIN )*4095 /(T_MAX  - T_MIN));

p  = dec2bin(position);
p  = [repmat('0', 1, 16-length(p)),p];
v  = dec2bin(velocity);
v  = [repmat('0', 1, 12-length(v)),v];
kp = dec2bin(K_p);
kp  = [repmat('0', 1, 12-length(kp)),kp];
kd = dec2bin(K_d);
kd  = [repmat('0', 1, 12-length(kd)),kd];
t  = dec2bin(T_ff);
t  = [repmat('0', 1, 12-length(t)),t];

B = repmat('0', 8, 8);

B(1,:) = p(1:8);
B(2,:) = p(9:16);
B(3,:) = v(1:8);
B(4,:) = [v(9:12),kp(1:4)];
B(5,:) = kp(5:12);
B(6,:) = kd(1:8);
B(7,:) = [kd(9:12),t(1:4)];
B(8,:) = t(5:12);

B  = bin2dec(B);

b = uint8(B);

== matlab function main_quad_rev5_31_315pm/ID3 Write Hip Data/floats -> bytes ==
  data: position input; b output uint8 size=8; velocity input; K_p input; K_d input; T_ff input
function b = fcn(position, velocity, K_p, K_d, T_ff)

P_MIN  =-95.5;  % [rad]
P_MAX  = 95.5;  % [rad]
V_MIN  =-45;    % [rad/s] 30 to 45
V_MAX  = 45;    % [rad/s]
KP_MIN = 0;     % [Nm/rad]
KP_MAX = 500;   % [Nm/rad]
KD_MIN = 0;     % [Nm*s/rad
KD_MAX = 5;     % [Nm*s/rad
T_MIN  =-18;    % [Nm]
T_MAX  = 18;    % [Nm]

position = floor((max(min(position,P_MAX) ,P_MIN)  - P_MIN )*65535/(P_MAX  - P_MIN));
velocity = floor((max(min(velocity,V_MAX) ,V_MIN)  - V_MIN )*4095 /(V_MAX  - V_MIN));
K_p      = floor((max(min(K_p     ,KP_MAX),KP_MIN) - KP_MIN)*4095 /(KP_MAX - KP_MIN));
K_d      = floor((max(min(K_d     ,V_MAX) ,V_MIN)  - KD_MIN)*4095 /(KD_MAX - KD_MIN));
T_ff     = floor((max(min(T_ff    ,V_MAX) ,V_MIN)  - T_MIN )*4095 /(T_MAX  - T_MIN));

p  = dec2bin(position);
p  = [repmat('0', 1, 16-length(p)),p];
v  = dec2bin(velocity);
v  = [repmat('0', 1, 12-length(v)),v];
kp = dec2bin(K_p);
kp  = [repmat('0', 1, 12-length(kp)),kp];
kd = dec2bin(K_d);
kd  = [repmat('0', 1, 12-length(kd)),kd];
t  = dec2bin(T_ff);
t  = [repmat('0', 1, 12-length(t)),t];

B = repmat('0', 8, 8);

B(1,:) = p(1:8);
B(2,:) = p(9:16);
B(3,:) = v(1:8);
B(4,:) = [v(9:12),kp(1:4)];
B(5,:) = kp(5:12);
B(6,:) = kd(1:8);
B(7,:) = [kd(9:12),t(1:4)];
B(8,:) = t(5:12);

B  = bin2dec(B);

b = uint8(B);

== matlab function main_quad_rev5_31_315pm/Danger Detector Function ==
  data: Pmux input; danger output
function danger = isDanger(Pmux)
    % Pmux position matrix radians
    %       [p(ID1),p(ID2),p(ID3),p(IDN)]

    
    p1Max = 2; 
    p1Min = -2;
    p2Max = 2;
    p2Min = -2;
    
    P1 = Pmux(1:2:end);
    P2 = Pmux(2:2:end);
       
    danger = 0;
    if((0<sum([P1>p1Max] + [P1<p1Min] - [P1<=-95.5])) || (0<sum([P2>p2Max] + [P2<p2Min] - [P2<=-95.5])))
    
%     if((0<sum([P1>p1Max] + [P1<p1Min])) || (0<sum([P2>p2Max] + [P2<p2Min])))
        danger = 1;
    end
